simulink model "memoire_avec_registre"  (R2014a)
settings: Solver=ode45  StartTime=0.0  StopTime=10.0  RelTol=1e-3
settings Model: Creator=elkhadiy  LastModifiedBy=elkhadiy

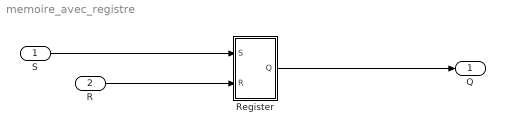
== system memoire_avec_registre ==
  S : Inport
  R : Inport  Port=2
  Register : Subsystem
  Q : Outport
  wires:
  S/1 -> Register/1(S)
  R/1 -> Register/2(R)
  Register/1(Q) -> Q/1

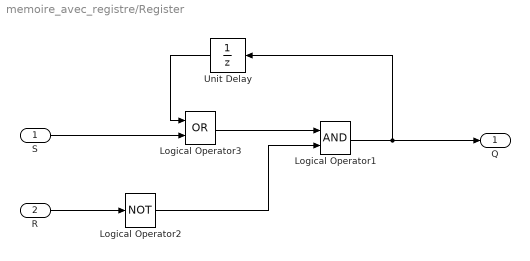
== system memoire_avec_registre/Register ==
  S : Inport
  R : Inport  Port=2
  Logical Operator1 : Logic  AllPortsSameDT=off  OutDataTypeStr=boolean
  Logical Operator2 : Logic  Operator=NOT  AllPortsSameDT=off  OutDataTypeStr=boolean
  Logical Operator3 : Logic  Operator=OR  AllPortsSameDT=off  OutDataTypeStr=boolean
  Unit Delay : UnitDelay  SampleTime=-1
  Q : Outport
  wires:
  Logical Operator1/1 -> Unit Delay/1, Q/1
  Unit Delay/1 -> Logical Operator3/1
  Logical Operator2/1 -> Logical Operator1/2
  Logical Operator3/1 -> Logical Operator1/1
  S/1 -> Logical Operator3/2
  R/1 -> Logical Operator2/1
